simulink model "serial_interface1"  (R2015a)
settings: Solver=ode3  StartTime=0.0  StopTime=0.5  FixedStep=0.001  RelTol=1e-3
values from neighbouring files (symbols this model uses):
  code = 11    [log_plot.m]
undefined symbols (not defined in the file or in its folder): LF, serial
libraries: simulink x3, instrumentlib x3
settings Model: Creator=rblan  LastModifiedBy=rblan
settings HardwareCC: ProdBitPerInt=16  ProdBitPerPointer=16  ProdLargestAtomicInteger=Integer  ProdLargestAtomicFloat=Float  ProdIntDivRoundTo=Zero  ProdEndianess=LittleEndian  ProdWordSize=16  ProdHWDeviceType=Microchip->dsPIC

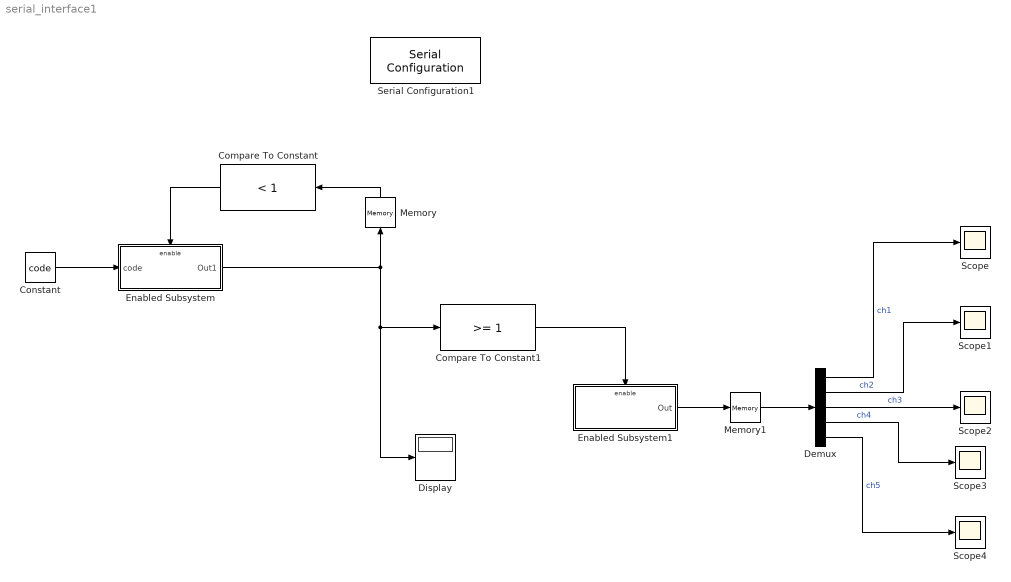
== system serial_interface1 ==
  Compare To Constant : simulink/Logic and Bit Operations/Compare To Constant  relop=<  const=1  OutDataTypeStr=boolean
  Compare To Constant1 : simulink/Logic and Bit Operations/Compare To Constant  relop=>=  const=1  OutDataTypeStr=boolean
  Constant : Constant  Value=code  SampleTime=0.001
  Demux : Demux  Outputs=5
  Display : Display
  Enabled Subsystem : Subsystem  TreatAsAtomicUnit=on
  Enabled Subsystem1 : Subsystem  TreatAsAtomicUnit=on
  Memory : Memory
  Memory1 : Memory
  Scope{,1..4} (5 alike) : Scope
      Scope settings: DataFormat=Structure
      Scope1 settings: DataFormat=Structure
      Scope2 settings: SaveName=ScopeData2  DataFormat=Structure
      Scope3 settings: SaveName=ScopeData3  DataFormat=Structure
      Scope4 settings: SaveName=ScopeData4  DataFormat=Structure
  Serial Configuration1 : instrumentlib/Serial Configuration  Priority=-200000  ComPortMenu=<Please select a port...>  ComPort=COM3  ObjConstructor=serial('COM3');  BaudRate=460800  DataBits=8  Parity=none  StopBits=1  FlowControl=none  Timeout=10  ByteOrder=BigEndian
  wires:
  Constant/1 -> Enabled Subsystem/1(code)
  Compare To Constant/1 -> Enabled Subsystem/Enable
  Memory/1 -> Compare To Constant/1
  Compare To Constant1/1 -> Enabled Subsystem1/Enable
  Enabled Subsystem1/1(Out) -> Memory1/1
  Demux/1 -> Scope/1  "ch1"
  Demux/2 -> Scope1/1  "ch2"
  Demux/3 -> Scope2/1  "ch3"
  Memory1/1 -> Demux/1
  Enabled Subsystem/1(Out1) -> Memory/1, Compare To Constant1/1, Display/1
  Demux/4 -> Scope3/1  "ch4"
  Demux/5 -> Scope4/1  "ch5"

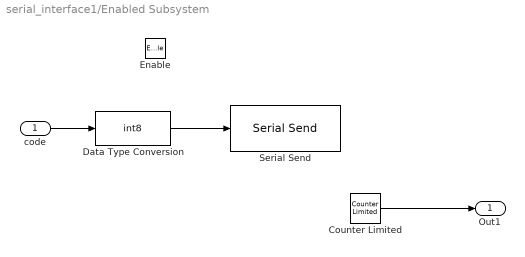
== system serial_interface1/Enabled Subsystem ==
  code : Inport
  Enable : EnablePort
  Counter Limited : simulink/Sources/Counter Limited  uplimit=2  tsamp=-1
  Data Type Conversion : DataTypeConversion  OutDataTypeStr=int8
  Serial Send : instrumentlib/Serial Send  ComPortMenu=COM3  ComPort=COM3  ObjConstructor=serial('COM3');  Terminator=<none>  EnableBlockingMode=off
  Out1 : Outport
  wires:
  Data Type Conversion/1 -> Serial Send/1
  code/1 -> Data Type Conversion/1
  Counter Limited/1 -> Out1/1

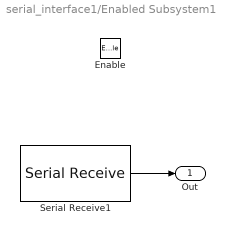
== system serial_interface1/Enabled Subsystem1 ==
  Enable : EnablePort
  Serial Receive1 : instrumentlib/Serial Receive  ComPortMenu=COM3  ComPort=COM3  ObjConstructor=serial('COM3');  Terminator=LF ('\n')  DataSize="[5  1]"  DataType=single  EnableBlockingMode=on  ActionDataUnavailable=Output last received value  CustomValue=0  SampleTime=0.001
  Out : Outport
  wires:
  Serial Receive1/1 -> Out/1
